simulink model "CF009A_GmOvrlStMgr"  (R2013b)
settings: Solver=FixedStepDiscrete  SolverMode=SingleTasking  StartTime=0.0  StopTime=1  FixedStep=0.002  RelTol=1e-3
values from neighbouring files (symbols this model uses):
  APASTACTV_CNT_U08 = DataDict.Constant    [CF009A_GmOvrlStMgr_DataDict.m]
  APASTCTRLAVL_CNT_U08 = DataDict.Constant    [CF009A_GmOvrlStMgr_DataDict.m]
  ARCHGLBPRM_2MILLISEC_SEC_F32 = DataDict.Constant    [CF009A_GmOvrlStMgr_DataDict.m]
  GmOvrlStMgrApaHwTqThd = DataDict.Calibration    [CF009A_GmOvrlStMgr_DataDict.m]
  GmOvrlStMgrApaHwTqTiThd = DataDict.Calibration    [CF009A_GmOvrlStMgr_DataDict.m]
  GmOvrlStMgrApaMfgEna = DataDict.Calibration    [CF009A_GmOvrlStMgr_DataDict.m]
  GmOvrlStMgrEscMfgEna = DataDict.Calibration    [CF009A_GmOvrlStMgr_DataDict.m]
  GmOvrlStMgrHaptcAmp = DataDict.Calibration    [CF009A_GmOvrlStMgr_DataDict.m]
  GmOvrlStMgrHaptcDurn = DataDict.Calibration    [CF009A_GmOvrlStMgr_DataDict.m]
  GmOvrlStMgrHaptcFrq = DataDict.Calibration    [CF009A_GmOvrlStMgr_DataDict.m]
  GmOvrlStMgrHaptcReactnTi = DataDict.Calibration    [CF009A_GmOvrlStMgr_DataDict.m]
  GmOvrlStMgrHaptcReqTiThd = DataDict.Calibration    [CF009A_GmOvrlStMgr_DataDict.m]
  GmOvrlStMgrHwAgTarLimr = DataDict.Calibration    [CF009A_GmOvrlStMgr_DataDict.m]
  GmOvrlStMgrLkaHwTqThd1 = DataDict.Calibration    [CF009A_GmOvrlStMgr_DataDict.m]
  GmOvrlStMgrLkaHwTqThd2 = DataDict.Calibration    [CF009A_GmOvrlStMgr_DataDict.m]
  GmOvrlStMgrLkaHwTqTiThd1 = DataDict.Calibration    [CF009A_GmOvrlStMgr_DataDict.m]
  GmOvrlStMgrLkaHwTqTiThd2 = DataDict.Calibration    [CF009A_GmOvrlStMgr_DataDict.m]
  GmOvrlStMgrLkaMfgEna = DataDict.Calibration    [CF009A_GmOvrlStMgr_DataDict.m]
  GmOvrlStMgrLoaMtgtnHaptcFbOffTi = DataDict.Calibration    [CF009A_GmOvrlStMgr_DataDict.m]
  GmOvrlStMgrLoaMtgtnHaptcFbOnTi = DataDict.Calibration    [CF009A_GmOvrlStMgr_DataDict.m]
  GmOvrlStMgrLoaMtgtnHaptcFbStrtOnTi = DataDict.Calibration    [CF009A_GmOvrlStMgr_DataDict.m]
  GmOvrlStMgrLoaMtgtnHaptcFbTqMax = DataDict.Calibration    [CF009A_GmOvrlStMgr_DataDict.m]
  GmOvrlStMgrLoaMtgtnHaptcFbTqMin = DataDict.Calibration    [CF009A_GmOvrlStMgr_DataDict.m]
  GmOvrlStMgrLoaMtgtnHaptcFbVehSpdMax = DataDict.Calibration    [CF009A_GmOvrlStMgr_DataDict.m]
  GmOvrlStMgrLoaMtgtnHaptcFbVehSpdMin = DataDict.Calibration    [CF009A_GmOvrlStMgr_DataDict.m]
  GmOvrlStMgrLoaMtgtnHaptcFrq = DataDict.Calibration    [CF009A_GmOvrlStMgr_DataDict.m]
  GmOvrlStMgrLoaMtgtnStrtHaptcAmp = DataDict.Calibration    [CF009A_GmOvrlStMgr_DataDict.m]
  GmOvrlStMgrLoaStIgnCntrThd = DataDict.Calibration    [CF009A_GmOvrlStMgr_DataDict.m]
  GmOvrlStMgrShiftLvrTiThd = DataDict.Calibration    [CF009A_GmOvrlStMgr_DataDict.m]
  GmOvrlStMgrStandStillThd = DataDict.Calibration    [CF009A_GmOvrlStMgr_DataDict.m]
  GmOvrlStMgrStandStillTiThd = DataDict.Calibration    [CF009A_GmOvrlStMgr_DataDict.m]
  HAPTCSTACTV_CNT_U08 = DataDict.Constant    [CF009A_GmOvrlStMgr_DataDict.m]
  HAPTCSTWAIT_CNT_U08 = DataDict.Constant    [CF009A_GmOvrlStMgr_DataDict.m]
  HWOSCNFRQMIN_HZ_F32 = DataDict.Constant    [CF009A_GmOvrlStMgr_DataDict.m]
  LKAFLTCNTRTHD_CNT_U08 = DataDict.Constant    [CF009A_GmOvrlStMgr_DataDict.m]
  LKAFLTTMRTHD_MILLISEC_U32 = DataDict.Constant    [CF009A_GmOvrlStMgr_DataDict.m]
  LKASTPRMNTFAILD_CNT_U08 = DataDict.Constant    [CF009A_GmOvrlStMgr_DataDict.m]
  LoaMtgtnThdExcdd = DataDict.NTC    [CF009A_GmOvrlStMgr_DataDict.m]
  MILLISECTO100MICROSECCNVN_CNT_U32 = DataDict.Constant    [CF009A_GmOvrlStMgr_DataDict.m]
  NODEBSTEP_CNT_U16 = DataDict.Constant    [CF009A_GmOvrlStMgr_DataDict.m]
undefined symbols (not defined in the file or in its folder): LoaSt1, NtcSts1, NVM_RequestResultType, SysSt1
libraries: simulink x13, Fil x6, NxtrNvM x4, NxtrLim x4, NxtrAbslt x3, NxtrSign x2, FixdToFloat x1, FloatToFixd x1, LnrIntrpn x1
(part 4 of 8)

== system CF009A_GmOvrlStMgr/GmOvrlStMgr/GmOvrlStMgrPer1/Inct_IgnCntr_Once/IgnCntr ==
  IgnCntrLcl : Inport  RequirementInfo={} %GIDa_40254b48_8d20_47a3_99f1_0af0fba286b0
  Action Port : ActionPort  InitializeStates=reset  ActionType=then
  Add : Sum
  Constant1 : Constant  Value=true  OutDataTypeStr=boolean
      settings: AttributesFormatString=%<OutDataTypeStr>
  Constant7 : Constant  Value=true  OutDataTypeStr=boolean
      settings: AttributesFormatString=%<OutDataTypeStr>
  Constant8 : Constant  OutDataTypeStr=Inherit: Inherit via back propagation
  CopyRight2 : Subsystem  Description=|  mask(Copyright Information){none=on}
      | Copyright info block.                                               
      |                                                                     
      | Place copyright information at the top of every subsystem in design.
      mask prompts: none "No parameters"
      mask help: Place copyright information at the top of every subsystem in design.
      mask Display:
      | NxtrConf = 'Nexteer Confidential';
      | 
      | sys = bdroot; %handle for the current model ("system")
      | first = get_param(sys,'Created');
      | if(isempty(first))
      |     first = datestr(now,'yyyy');
      | else
      |     first = first(end-3:end);  %year is last four digits
      | end
      | 
      | last = get_param(sys,'LastModifiedDate');
      | if isempty(last)
      |     last = datestr(now,'yyyy');
      | else
      |     last = last(end-3:end);
      | end
      | 
      | if strcmp(first,last)
      |     fprintf('%s -- Copyright %s Nexteer',NxtrConf,first)
      | else
      |     fprintf('%s -- %s%s- %s Nexteer',NxtrConf,char(169),first,last)
      | end
  Data Store Write7 : DataStoreWrite  DataStoreName=IgnCntrUpd
  Data Store Write9 : DataStoreWrite  DataStoreName=GmLoaIgnCntr
  GmLoaIgnCntr_Set Ram Block Status : NxtrNvM/Set Ram Block Status  FuncName=Set Ram Block Status  NvMBlockName=GmLoaIgnCntr  VoidFuncRtn=on  BlockChanged_DSN=NvMSRBS_BlockChanged  Return_DSN=NvMSRBS_Return
      settings: AttributesFormatString=%<FuncName>
  wires:
  Constant8/1 -> Add/2
  IgnCntrLcl/1 -> Add/1
  Add/1 -> Data Store Write9/1
  Constant7/1 -> Data Store Write7/1
  Constant1/1 -> GmLoaIgnCntr_Set Ram Block Status/1

== system CF009A_GmOvrlStMgr/GmOvrlStMgr/GmOvrlStMgrPer1/LKAIntv/CopyRight2 ==

== system CF009A_GmOvrlStMgr/GmOvrlStMgr/GmOvrlStMgrPer1/LKAIntv/HwTqLkaTqSignEqu ==
  Action Port : ActionPort  ActionType=then
  Constant13 : Constant  RequirementInfo={} %GIDa_343d1ac2_1708_4e02_a600_9208d3bcc3bc  Value=false  OutDataTypeStr=boolean
      settings: AttributesFormatString=%<OutDataTypeStr>
  CopyRight2 : Subsystem  Description=|  mask(Copyright Information){none=on}
      | Copyright info block.                                               
      |                                                                     
      | Place copyright information at the top of every subsystem in design.
      mask prompts: none "No parameters"
      mask help: Place copyright information at the top of every subsystem in design.
      mask Display:
      | NxtrConf = 'Nexteer Confidential';
      | 
      | sys = bdroot; %handle for the current model ("system")
      | first = get_param(sys,'Created');
      | first = first(end-3:end);  %year is last four digits
      | 
      | last = get_param(sys,'LastModifiedDate');
      | if isempty(last)
      |     last = datestr(now,'yyyy');
      | else
      |     last = last(end-3:end);
      | end
      | 
      | if strcmp(first,last)
      |     fprintf('%s -- Copyright %s Nexteer',NxtrConf,first)
      | else
      |     fprintf('%s -- %s%s- %s Nexteer',NxtrConf,char(169),first,last)
      | end
  Data Store Write1 : DataStoreWrite  DataStoreName=LkaIntvRefTi2
  Data Store Write9 : DataStoreWrite  DataStoreName=LkaIntvRefTi1
  GetRefTmr100MicroSec32bit : Subsystem
  GetRefTmr100MicroSec32bit_1 : Subsystem
  LKAIntv : Outport
  wires:
  Constant13/1 -> LKAIntv/1
  GetRefTmr100MicroSec32bit/1(RefTmr) -> Data Store Write9/1
  GetRefTmr100MicroSec32bit_1/1(RefTmr) -> Data Store Write1/1

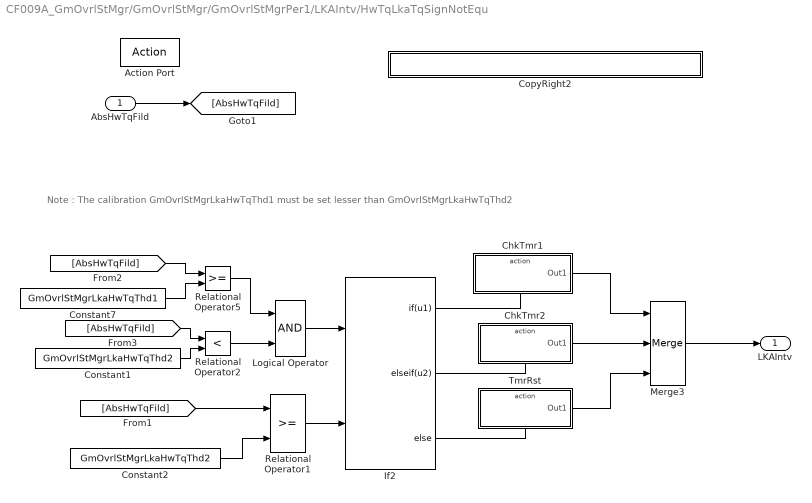
== system CF009A_GmOvrlStMgr/GmOvrlStMgr/GmOvrlStMgrPer1/LKAIntv/HwTqLkaTqSignNotEqu ==
  note: Note : The calibration GmOvrlStMgrLkaHwTqThd1 must be set lesser than GmOvrlStMgrLkaHwTqThd2
  AbsHwTqFild : Inport
  Action Port : ActionPort  ActionType=else
  ChkTmr1 : Subsystem  TreatAsAtomicUnit=on
  ChkTmr2 : Subsystem  TreatAsAtomicUnit=on
  Constant1 : Constant  Value=GmOvrlStMgrLkaHwTqThd2
  Constant2 : Constant  Value=GmOvrlStMgrLkaHwTqThd2
  Constant7 : Constant  Value=GmOvrlStMgrLkaHwTqThd1
  CopyRight2 : Subsystem  Description=|  mask(Copyright Information){none=on}
      | Copyright info block.                                               
      |                                                                     
      | Place copyright information at the top of every subsystem in design.
      mask prompts: none "No parameters"
      mask help: Place copyright information at the top of every subsystem in design.
      mask Display:
      | NxtrConf = 'Nexteer Confidential';
      | 
      | sys = bdroot; %handle for the current model ("system")
      | first = get_param(sys,'Created');
      | first = first(end-3:end);  %year is last four digits
      | 
      | last = get_param(sys,'LastModifiedDate');
      | if isempty(last)
      |     last = datestr(now,'yyyy');
      | else
      |     last = last(end-3:end);
      | end
      | 
      | if strcmp(first,last)
      |     fprintf('%s -- Copyright %s Nexteer',NxtrConf,first)
      | else
      |     fprintf('%s -- %s%s- %s Nexteer',NxtrConf,char(169),first,last)
      | end
  If2 : If  NumInputs=2  IfExpression=u1  ElseIfExpressions=u2
  Logical Operator : Logic  AllPortsSameDT=off  OutDataTypeStr=boolean
  Merge3 : Merge  Inputs=3
  Relational Operator1 : RelationalOperator  OutDataTypeStr=boolean
  Relational Operator2 : RelationalOperator  Operator=<  OutDataTypeStr=boolean
  Relational Operator5 : RelationalOperator  OutDataTypeStr=boolean
  TmrRst : Subsystem  TreatAsAtomicUnit=on
  LKAIntv : Outport
  wires:
  Logical Operator/1 -> If2/1
  Constant7/1 -> Relational Operator5/2
  [AbsHwTqFild] -> Relational Operator1/1
  Relational Operator1/1 -> If2/2
  Constant2/1 -> Relational Operator1/2
  If2/1 -> ChkTmr1/Action
  If2/2 -> ChkTmr2/Action
  If2/3 -> TmrRst/Action
  AbsHwTqFild/1 -> [AbsHwTqFild]
  [AbsHwTqFild] -> Relational Operator5/1
  ChkTmr2/1(Out1) -> Merge3/2
  ChkTmr1/1(Out1) -> Merge3/1
  TmrRst/1(Out1) -> Merge3/3
  Constant1/1 -> Relational Operator2/2
  [AbsHwTqFild] -> Relational Operator2/1
  Relational Operator5/1 -> Logical Operator/1
  Relational Operator2/1 -> Logical Operator/2
  Merge3/1 -> LKAIntv/1

== system CF009A_GmOvrlStMgr/GmOvrlStMgr/GmOvrlStMgrPer1/LkaCheck/CopyRight1 ==

== system CF009A_GmOvrlStMgr/GmOvrlStMgr/GmOvrlStMgrPer1/LkaCheck/CopyRight2 ==

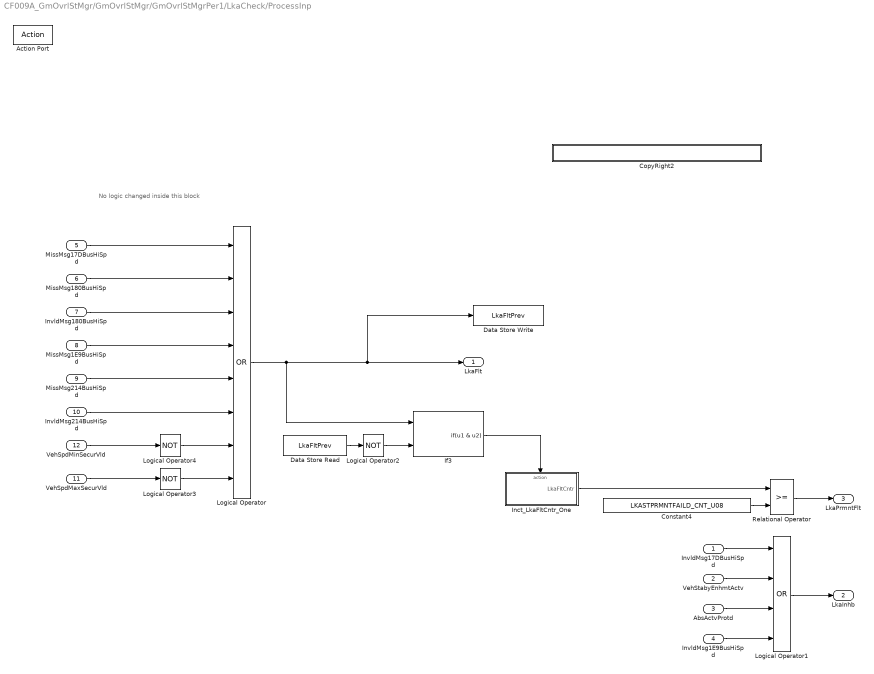
== system CF009A_GmOvrlStMgr/GmOvrlStMgr/GmOvrlStMgrPer1/LkaCheck/ProcessInp ==
  note: No logic changed inside this block
  InvldMsg17DBusHiSpd : Inport  RequirementInfo={} %GIDa_ab38f364_fb54_43ac_97fb_df178091b6c1
  VehStabyEnhmtActv : Inport  RequirementInfo={} %GIDa_14faf567_e873_4922_a66e_aab04f66d7c3  Port=2
  AbsActvProtd : Inport  RequirementInfo={} %GIDa_a55d01c1_013b_4525_9432_b498c288d3b3  Port=3
  InvldMsg1E9BusHiSpd : Inport  RequirementInfo={} %GIDa_3ed3612c_6ee8_4a1a_b952_8a9e955ddcf1  Port=4
  MissMsg17DBusHiSpd : Inport  RequirementInfo={} %GIDa_e64a72e9_2517_49f8_a6e5_489273597452  Port=5
  MissMsg180BusHiSpd : Inport  RequirementInfo={} %GIDa_2fabbd9a_4f5e_4808_82cc_2e9f3cd02a49  Port=6
  InvldMsg180BusHiSpd : Inport  RequirementInfo={} %GIDa_322da83d_5a43_4b7c_bcd7_98015d045729  Port=7
  MissMsg1E9BusHiSpd : Inport  RequirementInfo={} %GIDa_13222ae9_8796_4dca_b882_a83b9d93d3cb  Port=8
  MissMsg214BusHiSpd : Inport  RequirementInfo={} %GIDa_1bf44673_30db_49ae_bdac_03d5de220bff  Port=9
  InvldMsg214BusHiSpd : Inport  RequirementInfo={} %GIDa_9d83abc3_8b94_4471_9b6e_3a35c366fb39  Port=10
  VehSpdMaxSecurVld : Inport  Port=11
  VehSpdMinSecurVld : Inport  Port=12
  Action Port : ActionPort  ActionType=then
  Constant4 : Constant  RequirementInfo={} %GIDa_94974dc5_adaa_4b71_913a_ea3d1a9969a7  Value=LKASTPRMNTFAILD_CNT_U08
  CopyRight2 : Subsystem  Description=|  mask(Copyright Information){none=on}
      | Copyright info block.                                               
      |                                                                     
      | Place copyright information at the top of every subsystem in design.
      mask prompts: none "No parameters"
      mask help: Place copyright information at the top of every subsystem in design.
      mask Display:
      | NxtrConf = 'Nexteer Confidential';
      | 
      | sys = bdroot; %handle for the current model ("system")
      | first = get_param(sys,'Created');
      | if(isempty(first))
      |     first = datestr(now,'yyyy');
      | else
      |     first = first(end-3:end);  %year is last four digits
      | end
      | 
      | last = get_param(sys,'LastModifiedDate');
      | if isempty(last)
      |     last = datestr(now,'yyyy');
      | else
      |     last = last(end-3:end);
      | end
      | 
      | if strcmp(first,last)
      |     fprintf('%s -- Copyright %s Nexteer',NxtrConf,first)
      | else
      |     fprintf('%s -- %s%s- %s Nexteer',NxtrConf,char(169),first,last)
      | end
  Data Store Read : DataStoreRead  Priority=1  DataStoreName=LkaFltPrev
      settings: AttributesFormatString=Priority: %<Priority>
  Data Store Write : DataStoreWrite  Priority=2  DataStoreName=LkaFltPrev
      settings: AttributesFormatString=Priority: %<Priority>
  If3 : If  NumInputs=2  IfExpression=u1 & u2  ShowElse=off
  Inct_LkaFltCntr_One : Subsystem
  Logical Operator : Logic  Operator=OR  Inputs=8  AllPortsSameDT=off  OutDataTypeStr=boolean
  Logical Operator1 : Logic  Operator=OR  Inputs=4  AllPortsSameDT=off  OutDataTypeStr=boolean
  Logical Operator2 : Logic  Operator=NOT  AllPortsSameDT=off  OutDataTypeStr=boolean
  Logical Operator3 : Logic  Operator=NOT  AllPortsSameDT=off  OutDataTypeStr=boolean
  Logical Operator4 : Logic  Operator=NOT  AllPortsSameDT=off  OutDataTypeStr=boolean
  Relational Operator : RelationalOperator  OutDataTypeStr=boolean
  LkaFlt : Outport
  LkaInhb : Outport  Port=2
  LkaPrmntFlt : Outport  Port=3
  wires:
  Relational Operator/1 -> LkaPrmntFlt/1
  Logical Operator1/1 -> LkaInhb/1
  Constant4/1 -> Relational Operator/2
  MissMsg17DBusHiSpd/1 -> Logical Operator/1
  MissMsg180BusHiSpd/1 -> Logical Operator/2
  InvldMsg180BusHiSpd/1 -> Logical Operator/3
  MissMsg1E9BusHiSpd/1 -> Logical Operator/4
  MissMsg214BusHiSpd/1 -> Logical Operator/5
  InvldMsg214BusHiSpd/1 -> Logical Operator/6
  InvldMsg17DBusHiSpd/1 -> Logical Operator1/1
  VehStabyEnhmtActv/1 -> Logical Operator1/2
  AbsActvProtd/1 -> Logical Operator1/3
  InvldMsg1E9BusHiSpd/1 -> Logical Operator1/4
  Logical Operator/1 -> If3/1, Data Store Write/1, LkaFlt/1
  If3/1 -> Inct_LkaFltCntr_One/Action
  Inct_LkaFltCntr_One/1(LkaFltCntr) -> Relational Operator/1
  VehSpdMinSecurVld/1 -> Logical Operator4/1
  VehSpdMaxSecurVld/1 -> Logical Operator3/1
  Data Store Read/1 -> Logical Operator2/1
  Logical Operator2/1 -> If3/2
  Logical Operator3/1 -> Logical Operator/8
  Logical Operator4/1 -> Logical Operator/7

== system CF009A_GmOvrlStMgr/GmOvrlStMgr/GmOvrlStMgrPer1/LkaCheck/SetDefVal ==
  Action Port : ActionPort  ActionType=else
  Constant1 : Constant  Value=0  OutDataTypeStr=boolean
      settings: AttributesFormatString=%<OutDataTypeStr>
  Constant2 : Constant  Value=0  OutDataTypeStr=boolean
      settings: AttributesFormatString=%<OutDataTypeStr>
  Constant6 : Constant  Value=0  OutDataTypeStr=boolean
      settings: AttributesFormatString=%<OutDataTypeStr>
  CopyRight2 : Subsystem  Description=|  mask(Copyright Information){none=on}
      | Copyright info block.                                               
      |                                                                     
      | Place copyright information at the top of every subsystem in design.
      mask prompts: none "No parameters"
      mask help: Place copyright information at the top of every subsystem in design.
      mask Display:
      | NxtrConf = 'Nexteer Confidential';
      | 
      | sys = bdroot; %handle for the current model ("system")
      | first = get_param(sys,'Created');
      | if(isempty(first))
      |     first = datestr(now,'yyyy');
      | else
      |     first = first(end-3:end);  %year is last four digits
      | end
      | 
      | last = get_param(sys,'LastModifiedDate');
      | if isempty(last)
      |     last = datestr(now,'yyyy');
      | else
      |     last = last(end-3:end);
      | end
      | 
      | if strcmp(first,last)
      |     fprintf('%s -- Copyright %s Nexteer',NxtrConf,first)
      | else
      |     fprintf('%s -- %s%s- %s Nexteer',NxtrConf,char(169),first,last)
      | end
  LkaFlt : Outport
  LkaInhb : Outport  Port=2
  LkaPrmntFlt : Outport  Port=3
  wires:
  Constant6/1 -> LkaFlt/1
  Constant1/1 -> LkaInhb/1
  Constant2/1 -> LkaPrmntFlt/1

== system CF009A_GmOvrlStMgr/GmOvrlStMgr/GmOvrlStMgrPer1/LkaCheck/TmrElpdDetn ==
  LkaFltRefTmr : Inport
  Constant : Constant  Value=LKAFLTTMRTHD_MILLISEC_U32
  Constant1 : Constant  Value=MILLISECTO100MICROSECCNVN_CNT_U32
  CopyRight2 : Subsystem  Description=|  mask(Copyright Information){none=on}
      | Copyright info block.                                               
      |                                                                     
      | Place copyright information at the top of every subsystem in design.
      mask prompts: none "No parameters"
      mask help: Place copyright information at the top of every subsystem in design.
      mask Display:
      | NxtrConf = 'Nexteer Confidential';
      | 
      | sys = bdroot; %handle for the current model ("system")
      | first = get_param(sys,'Created');
      | if(isempty(first))
      |     first = datestr(now,'yyyy');
      | else
      |     first = first(end-3:end);  %year is last four digits
      | end
      | 
      | last = get_param(sys,'LastModifiedDate');
      | if isempty(last)
      |     last = datestr(now,'yyyy');
      | else
      |     last = last(end-3:end);
      | end
      | 
      | if strcmp(first,last)
      |     fprintf('%s -- Copyright %s Nexteer',NxtrConf,first)
      | else
      |     fprintf('%s -- %s%s- %s Nexteer',NxtrConf,char(169),first,last)
      | end
  GetTiSpan100MicroSec32bit : Subsystem
  Product : Product
  Relational Operator : RelationalOperator  OutDataTypeStr=boolean
  TiElpd : Outport
  wires:
  LkaFltRefTmr/1 -> GetTiSpan100MicroSec32bit/1(RefTmr)
  GetTiSpan100MicroSec32bit/1(TiSpan) -> Relational Operator/1
  Product/1 -> Relational Operator/2
  Constant/1 -> Product/1
  Constant1/1 -> Product/2
  Relational Operator/1 -> TiElpd/1

== system CF009A_GmOvrlStMgr/GmOvrlStMgr/GmOvrlStMgrPer1/LoaStLimdOrSwBasdMtgtn/CopyRight2 ==

== system CF009A_GmOvrlStMgr/GmOvrlStMgr/GmOvrlStMgrPer1/LoaStLimdOrSwBasdMtgtn/Set_false_LoaStLimdOrSwBasdMtgtn ==
  Action Port : ActionPort  ActionType=else
  Constant2 : Constant  Value=false  OutDataTypeStr=boolean
      settings: AttributesFormatString=%<OutDataTypeStr>
  CopyRight2 : Subsystem  Description=|  mask(Copyright Information){none=on}
      | Copyright info block.                                               
      |                                                                     
      | Place copyright information at the top of every subsystem in design.
      mask prompts: none "No parameters"
      mask help: Place copyright information at the top of every subsystem in design.
      mask Display:
      | NxtrConf = 'Nexteer Confidential';
      | 
      | sys = bdroot; %handle for the current model ("system")
      | first = get_param(sys,'Created');
      | if(isempty(first))
      |     first = datestr(now,'yyyy');
      | else
      |     first = first(end-3:end);  %year is last four digits
      | end
      | 
      | last = get_param(sys,'LastModifiedDate');
      | if isempty(last)
      |     last = datestr(now,'yyyy');
      | else
      |     last = last(end-3:end);
      | end
      | 
      | if strcmp(first,last)
      |     fprintf('%s -- Copyright %s Nexteer',NxtrConf,first)
      | else
      |     fprintf('%s -- %s%s- %s Nexteer',NxtrConf,char(169),first,last)
      | end
  LoaStLimdOrSwBasdMtgtn : Outport
  wires:
  Constant2/1 -> LoaStLimdOrSwBasdMtgtn/1

== system CF009A_GmOvrlStMgr/GmOvrlStMgr/GmOvrlStMgrPer1/LoaStLimdOrSwBasdMtgtn/Set_true_LoaStLimdOrSwBasdMtgtn ==
  Action Port : ActionPort  ActionType=then
  Constant2 : Constant  Value=true  OutDataTypeStr=boolean
      settings: AttributesFormatString=%<OutDataTypeStr>
  CopyRight2 : Subsystem  Description=|  mask(Copyright Information){none=on}
      | Copyright info block.                                               
      |                                                                     
      | Place copyright information at the top of every subsystem in design.
      mask prompts: none "No parameters"
      mask help: Place copyright information at the top of every subsystem in design.
      mask Display:
      | NxtrConf = 'Nexteer Confidential';
      | 
      | sys = bdroot; %handle for the current model ("system")
      | first = get_param(sys,'Created');
      | if(isempty(first))
      |     first = datestr(now,'yyyy');
      | else
      |     first = first(end-3:end);  %year is last four digits
      | end
      | 
      | last = get_param(sys,'LastModifiedDate');
      | if isempty(last)
      |     last = datestr(now,'yyyy');
      | else
      |     last = last(end-3:end);
      | end
      | 
      | if strcmp(first,last)
      |     fprintf('%s -- Copyright %s Nexteer',NxtrConf,first)
      | else
      |     fprintf('%s -- %s%s- %s Nexteer',NxtrConf,char(169),first,last)
      | end
  LoaStLimdOrSwBasdMtgtn : Outport
  wires:
  Constant2/1 -> LoaStLimdOrSwBasdMtgtn/1

== system CF009A_GmOvrlStMgr/GmOvrlStMgr/GmOvrlStMgrPer1/SysStNotOperate_TqOscnDi_AmpZero_FrqMin/CopyRight2 ==

== system CF009A_GmOvrlStMgr/GmOvrlStMgr/GmOvrlStMgrPer1/SysStOperate/Chk_LoaSt_IgnCntr_ AtStartUp ==
  IgnCntrLcl : Inport  RequirementInfo={} %GIDa_e8697a3d_ab56_4bb3_bef2_1b8a01945d63
  LoaStLimdOrSwBasdMtgtn : Inport  RequirementInfo={} %GIDa_6f19b0cf_19ed_4211_a8d1_72361d5bd862  Port=2
  Action Port : ActionPort  ActionType=then
  Constant5 : Constant  Value=GmOvrlStMgrLoaStIgnCntrThd
  CopyRight2 : Subsystem  Description=|  mask(Copyright Information){none=on}
      | Copyright info block.                                               
      |                                                                     
      | Place copyright information at the top of every subsystem in design.
      mask prompts: none "No parameters"
      mask help: Place copyright information at the top of every subsystem in design.
      mask Display:
      | NxtrConf = 'Nexteer Confidential';
      | 
      | sys = bdroot; %handle for the current model ("system")
      | first = get_param(sys,'Created');
      | if(isempty(first))
      |     first = datestr(now,'yyyy');
      | else
      |     first = first(end-3:end);  %year is last four digits
      | end
      | 
      | last = get_param(sys,'LastModifiedDate');
      | if isempty(last)
      |     last = datestr(now,'yyyy');
      | else
      |     last = last(end-3:end);
      | end
      | 
      | if strcmp(first,last)
      |     fprintf('%s -- Copyright %s Nexteer',NxtrConf,first)
      | else
      |     fprintf('%s -- %s%s- %s Nexteer',NxtrConf,char(169),first,last)
      | end
  HaptcFbOn : Subsystem  TreatAsAtomicUnit=on
  If4 : If  NumInputs=2  IfExpression=u1&u2
  Merge1 : Merge
  Merge2 : Merge
  Merge3 : Merge
  Relational Operator5 : RelationalOperator  Operator=<  OutDataTypeStr=boolean
  Set_True_LoaStAlreadyChk_HaptcFbOff : Subsystem  TreatAsAtomicUnit=on
  HaptcFbEn : Outport
  HwOscnMotAmp : Outport  RequirementInfo={} %GIDa_94979410_e9f4_4c1d_b419_ebbe160cd395  Port=2
  HwOscnFrq : Outport  RequirementInfo={} %GIDa_7e58c67f_3cab_4a1d_80f1_5b93bb1627c0  Port=3
  wires:
  If4/1 -> HaptcFbOn/Action
  If4/2 -> Set_True_LoaStAlreadyChk_HaptcFbOff/Action
  HaptcFbOn/2(HwOscnMotAmp) -> Merge1/1
  HaptcFbOn/1(HaptcFbEn) -> Merge2/1
  HaptcFbOn/3(HwOscnFrq) -> Merge3/1
  Set_True_LoaStAlreadyChk_HaptcFbOff/1(HwOscnEna) -> Merge2/2
  Set_True_LoaStAlreadyChk_HaptcFbOff/3(HwOscnFrq) -> Merge3/2
  Set_True_LoaStAlreadyChk_HaptcFbOff/2(HwOscnMotAmp) -> Merge1/2
  Merge2/1 -> HaptcFbEn/1
  Merge3/1 -> HwOscnFrq/1
  Merge1/1 -> HwOscnMotAmp/1
  Constant5/1 -> Relational Operator5/2
  IgnCntrLcl/1 -> Relational Operator5/1
  Relational Operator5/1 -> If4/1
  LoaStLimdOrSwBasdMtgtn/1 -> If4/2

== system CF009A_GmOvrlStMgr/GmOvrlStMgr/GmOvrlStMgrPer1/SysStOperate/CopyRight2 ==

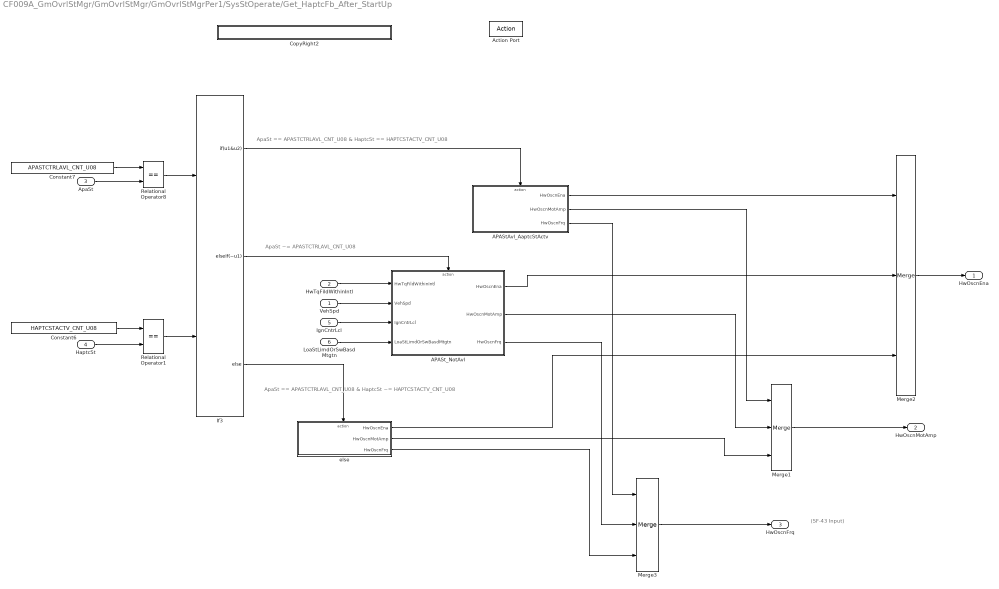
== system CF009A_GmOvrlStMgr/GmOvrlStMgr/GmOvrlStMgrPer1/SysStOperate/Get_HaptcFb_After_StartUp ==
  note: ApaSt == APASTCTRLAVL_CNT_U08 & HaptcSt ~= HAPTCSTACTV_CNT_U08
  note: ApaSt ~= APASTCTRLAVL_CNT_U08
  note: ApaSt == APASTCTRLAVL_CNT_U08 & HaptcSt == HAPTCSTACTV_CNT_U08
  note: (SF-43 Input)
  VehSpd : Inport  RequirementInfo={} %GIDa_a5829b81_07ba_4c64_8787_8fc04ee14cfd
  HwTqFildWithinIntl : Inport  RequirementInfo={} %GIDa_e61ff016_f3ba_4ff0_a83d_54857dcede2c  Port=2
  ApaSt : Inport  RequirementInfo={} %GIDa_e54ff0fb_14e3_45e1_9566_d1512fd62416  Port=3
  HaptcSt : Inport  RequirementInfo={} %GIDa_ab8a4f54_44b6_4424_b05e_8238140c4b6c  Port=4
  IgnCntrLcl : Inport  RequirementInfo={} %GIDa_b0910f28_8214_48fc_9951_e54f19ad46d2  Port=5
  LoaStLimdOrSwBasdMtgtn : Inport  RequirementInfo={} %GIDa_58f7fd75_e089_4fe4_9a52_37c69388915c  Port=6
  Action Port : ActionPort  ActionType=else
  APAStAvl_AaptcStActv : Subsystem
  APASt_NotAvl : Subsystem
  Constant6 : Constant  RequirementInfo={} %GIDa_58d35ea2_589d_40a1_bd0e_f64c7e93a79e  Value=HAPTCSTACTV_CNT_U08
  Constant7 : Constant  Value=APASTCTRLAVL_CNT_U08
  CopyRight2 : Subsystem  Description=|  mask(Copyright Information){none=on}
      | Copyright info block.                                               
      |                                                                     
      | Place copyright information at the top of every subsystem in design.
      mask prompts: none "No parameters"
      mask help: Place copyright information at the top of every subsystem in design.
      mask Display:
      | NxtrConf = 'Nexteer Confidential';
      | 
      | sys = bdroot; %handle for the current model ("system")
      | first = get_param(sys,'Created');
      | if(isempty(first))
      |     first = datestr(now,'yyyy');
      | else
      |     first = first(end-3:end);  %year is last four digits
      | end
      | 
      | last = get_param(sys,'LastModifiedDate');
      | if isempty(last)
      |     last = datestr(now,'yyyy');
      | else
      |     last = last(end-3:end);
      | end
      | 
      | if strcmp(first,last)
      |     fprintf('%s -- Copyright %s Nexteer',NxtrConf,first)
      | else
      |     fprintf('%s -- %s%s- %s Nexteer',NxtrConf,char(169),first,last)
      | end
  If3 : If  NumInputs=2  IfExpression=u1&u2  ElseIfExpressions=~u1
  Merge1 : Merge  Inputs=3
  Merge2 : Merge  Inputs=3
  Merge3 : Merge  Inputs=3
  Relational Operator1 : RelationalOperator  Operator===  OutDataTypeStr=boolean
  Relational Operator8 : RelationalOperator  Operator===  OutDataTypeStr=boolean
  else : Subsystem
  HwOscnEna : Outport  RequirementInfo={} %GIDa_60abaf6a_645d_41f4_bc17_5a7267f09745
  HwOscnMotAmp : Outport  RequirementInfo={} %GIDa_33c54218_d95c_4bd4_ac09_6c51a9d1e98a  Port=2
  HwOscnFrq : Outport  RequirementInfo={} %GIDa_08ffb019_6499_48c1_85d5_d35ae98c4cad  Port=3
  wires:
  VehSpd/1 -> APASt_NotAvl/2(VehSpd)
  Relational Operator1/1 -> If3/2
  Constant6/1 -> Relational Operator1/1
  Relational Operator8/1 -> If3/1
  If3/1 -> APAStAvl_AaptcStActv/Action
  If3/3 -> else/Action
  If3/2 -> APASt_NotAvl/Action
  Merge1/1 -> HwOscnMotAmp/1
  Merge3/1 -> HwOscnFrq/1
  APAStAvl_AaptcStActv/1(HwOscnEna) -> Merge2/1
  APASt_NotAvl/1(HwOscnEna) -> Merge2/2
  else/1(HwOscnEna) -> Merge2/3
  APAStAvl_AaptcStActv/2(HwOscnMotAmp) -> Merge1/1
  APASt_NotAvl/2(HwOscnMotAmp) -> Merge1/2
  else/2(HwOscnMotAmp) -> Merge1/3
  APAStAvl_AaptcStActv/3(HwOscnFrq) -> Merge3/1
  APASt_NotAvl/3(HwOscnFrq) -> Merge3/2
  else/3(HwOscnFrq) -> Merge3/3
  Merge2/1 -> HwOscnEna/1
  HwTqFildWithinIntl/1 -> APASt_NotAvl/1(HwTqFildWithinIntl)
  HaptcSt/1 -> Relational Operator1/2
  Constant7/1 -> Relational Operator8/1
  ApaSt/1 -> Relational Operator8/2
  IgnCntrLcl/1 -> APASt_NotAvl/3(IgnCntrLcl)
  LoaStLimdOrSwBasdMtgtn/1 -> APASt_NotAvl/4(LoaStLimdOrSwBasdMtgtn)

== system CF009A_GmOvrlStMgr/GmOvrlStMgr/GmOvrlStMgrPer1/Timer for HwHaptcEna/CopyRight2 ==

== system CF009A_GmOvrlStMgr/GmOvrlStMgr/GmOvrlStMgrPer1/Timer for HwHaptcEna/If Action Subsystem ==
  Action Port : ActionPort  ActionType=then
  Constant : Constant  Value=0  OutDataTypeStr=single
  CopyRight2 : Subsystem  Description=|  mask(Copyright Information){none=on}
      | Copyright info block.                                               
      |                                                                     
      | Place copyright information at the top of every subsystem in design.
      mask prompts: none "No parameters"
      mask help: Place copyright information at the top of every subsystem in design.
      mask Display:
      | NxtrConf = 'Nexteer Confidential';
      | 
      | sys = bdroot; %handle for the current model ("system")
      | first = get_param(sys,'Created');
      | if(isempty(first))
      |     first = datestr(now,'yyyy');
      | else
      |     first = first(end-3:end);  %year is last four digits
      | end
      | 
      | last = get_param(sys,'LastModifiedDate');
      | if isempty(last)
      |     last = datestr(now,'yyyy');
      | else
      |     last = last(end-3:end);
      | end
      | 
      | if strcmp(first,last)
      |     fprintf('%s -- Copyright %s Nexteer',NxtrConf,first)
      | else
      |     fprintf('%s -- %s%s- %s Nexteer',NxtrConf,char(169),first,last)
      | end
  Data Store Write : DataStoreWrite  DataStoreName=PrevHaptcReqRefTi
  Data Type Conversion : DataTypeConversion  OutDataTypeStr=uint32
  GetRefTmr100MicroSec32bit : Subsystem
  Out : Outport
  wires:
  Constant/1 -> Data Type Conversion/1
  GetRefTmr100MicroSec32bit/1(RefTmr) -> Data Store Write/1
  Data Type Conversion/1 -> Out/1

== system CF009A_GmOvrlStMgr/GmOvrlStMgr/GmOvrlStMgrPer1/Timer for HwHaptcEna/If Action Subsystem1 ==
  In1 : Inport
  Action Port : ActionPort  ActionType=else
  CopyRight2 : Subsystem  Description=|  mask(Copyright Information){none=on}
      | Copyright info block.                                               
      |                                                                     
      | Place copyright information at the top of every subsystem in design.
      mask prompts: none "No parameters"
      mask help: Place copyright information at the top of every subsystem in design.
      mask Display:
      | NxtrConf = 'Nexteer Confidential';
      | 
      | sys = bdroot; %handle for the current model ("system")
      | first = get_param(sys,'Created');
      | if(isempty(first))
      |     first = datestr(now,'yyyy');
      | else
      |     first = first(end-3:end);  %year is last four digits
      | end
      | 
      | last = get_param(sys,'LastModifiedDate');
      | if isempty(last)
      |     last = datestr(now,'yyyy');
      | else
      |     last = last(end-3:end);
      | end
      | 
      | if strcmp(first,last)
      |     fprintf('%s -- Copyright %s Nexteer',NxtrConf,first)
      | else
      |     fprintf('%s -- %s%s- %s Nexteer',NxtrConf,char(169),first,last)
      | end
  Out1 : Outport
  wires:
  In1/1 -> Out1/1

== system CF009A_GmOvrlStMgr/GmOvrlStMgr/GmOvrlStMgrPer1/Timer for HwHaptcEna/If Action Subsystem2 ==
  Action Port : ActionPort  ActionType=elseif
  CopyRight2 : Subsystem  Description=|  mask(Copyright Information){none=on}
      | Copyright info block.                                               
      |                                                                     
      | Place copyright information at the top of every subsystem in design.
      mask prompts: none "No parameters"
      mask help: Place copyright information at the top of every subsystem in design.
      mask Display:
      | NxtrConf = 'Nexteer Confidential';
      | 
      | sys = bdroot; %handle for the current model ("system")
      | first = get_param(sys,'Created');
      | if(isempty(first))
      |     first = datestr(now,'yyyy');
      | else
      |     first = first(end-3:end);  %year is last four digits
      | end
      | 
      | last = get_param(sys,'LastModifiedDate');
      | if isempty(last)
      |     last = datestr(now,'yyyy');
      | else
      |     last = last(end-3:end);
      | end
      | 
      | if strcmp(first,last)
      |     fprintf('%s -- Copyright %s Nexteer',NxtrConf,first)
      | else
      |     fprintf('%s -- %s%s- %s Nexteer',NxtrConf,char(169),first,last)
      | end
  Data Store Read : DataStoreRead  DataStoreName=PrevHaptcReqRefTi
  GetTiSpan100MicroSec32bit1 : Subsystem
  Out1 : Outport
  wires:
  GetTiSpan100MicroSec32bit1/1(TiSpan) -> Out1/1
  Data Store Read/1 -> GetTiSpan100MicroSec32bit1/1(RefTmr)

== system CF009A_GmOvrlStMgr/GmOvrlStMgr/GmOvrlStMgrPer1/Timer for ShiftLvrRvs/CopyRight2 ==

== system CF009A_GmOvrlStMgr/GmOvrlStMgr/GmOvrlStMgrPer1/Timer for ShiftLvrRvs/If Action Subsystem ==
  Action Port : ActionPort  ActionType=then
  Constant : Constant  Value=0  OutDataTypeStr=single
  CopyRight2 : Subsystem  Description=|  mask(Copyright Information){none=on}
      | Copyright info block.                                               
      |                                                                     
      | Place copyright information at the top of every subsystem in design.
      mask prompts: none "No parameters"
      mask help: Place copyright information at the top of every subsystem in design.
      mask Display:
      | NxtrConf = 'Nexteer Confidential';
      | 
      | sys = bdroot; %handle for the current model ("system")
      | first = get_param(sys,'Created');
      | first = first(end-3:end);  %year is last four digits
      | 
      | last = get_param(sys,'LastModifiedDate');
      | if isempty(last)
      |     last = datestr(now,'yyyy');
      | else
      |     last = last(end-3:end);
      | end
      | 
      | if strcmp(first,last)
      |     fprintf('%s -- Copyright %s Nexteer',NxtrConf,first)
      | else
      |     fprintf('%s -- %s%s- %s Nexteer',NxtrConf,char(169),first,last)
      | end
  Data Store Write : DataStoreWrite  DataStoreName=PrevShiftLvrRvsRefTi
  Data Type Conversion : DataTypeConversion  OutDataTypeStr=uint32
  GetRefTmr100MicroSec32bit : Subsystem
  Out : Outport
  wires:
  Constant/1 -> Data Type Conversion/1
  GetRefTmr100MicroSec32bit/1(RefTmr) -> Data Store Write/1
  Data Type Conversion/1 -> Out/1

== system CF009A_GmOvrlStMgr/GmOvrlStMgr/GmOvrlStMgrPer1/Timer for ShiftLvrRvs/If Action Subsystem1 ==
  In1 : Inport
  Action Port : ActionPort  ActionType=else
  CopyRight2 : Subsystem  Description=|  mask(Copyright Information){none=on}
      | Copyright info block.                                               
      |                                                                     
      | Place copyright information at the top of every subsystem in design.
      mask prompts: none "No parameters"
      mask help: Place copyright information at the top of every subsystem in design.
      mask Display:
      | NxtrConf = 'Nexteer Confidential';
      | 
      | sys = bdroot; %handle for the current model ("system")
      | first = get_param(sys,'Created');
      | first = first(end-3:end);  %year is last four digits
      | 
      | last = get_param(sys,'LastModifiedDate');
      | if isempty(last)
      |     last = datestr(now,'yyyy');
      | else
      |     last = last(end-3:end);
      | end
      | 
      | if strcmp(first,last)
      |     fprintf('%s -- Copyright %s Nexteer',NxtrConf,first)
      | else
      |     fprintf('%s -- %s%s- %s Nexteer',NxtrConf,char(169),first,last)
      | end
  Out1 : Outport
  wires:
  In1/1 -> Out1/1

== system CF009A_GmOvrlStMgr/GmOvrlStMgr/GmOvrlStMgrPer1/Timer for ShiftLvrRvs/If Action Subsystem2 ==
  Action Port : ActionPort  ActionType=elseif
  CopyRight2 : Subsystem  Description=|  mask(Copyright Information){none=on}
      | Copyright info block.                                               
      |                                                                     
      | Place copyright information at the top of every subsystem in design.
      mask prompts: none "No parameters"
      mask help: Place copyright information at the top of every subsystem in design.
      mask Display:
      | NxtrConf = 'Nexteer Confidential';
      | 
      | sys = bdroot; %handle for the current model ("system")
      | first = get_param(sys,'Created');
      | first = first(end-3:end);  %year is last four digits
      | 
      | last = get_param(sys,'LastModifiedDate');
      | if isempty(last)
      |     last = datestr(now,'yyyy');
      | else
      |     last = last(end-3:end);
      | end
      | 
      | if strcmp(first,last)
      |     fprintf('%s -- Copyright %s Nexteer',NxtrConf,first)
      | else
      |     fprintf('%s -- %s%s- %s Nexteer',NxtrConf,char(169),first,last)
      | end
  Data Store Read : DataStoreRead  DataStoreName=PrevShiftLvrRvsRefTi
  GetTiSpan100MicroSec32bit1 : Subsystem
  Out : Outport
  wires:
  GetTiSpan100MicroSec32bit1/1(TiSpan) -> Out/1
  Data Store Read/1 -> GetTiSpan100MicroSec32bit1/1(RefTmr)

== system CF009A_GmOvrlStMgr/GmOvrlStMgr/GmOvrlStMgrPer1/Timer for VehStandStill/CopyRight2 ==

== system CF009A_GmOvrlStMgr/GmOvrlStMgr/GmOvrlStMgrPer1/Timer for VehStandStill/If Action Subsystem ==
  Action Port : ActionPort  ActionType=then
  Constant : Constant  Value=0  OutDataTypeStr=single
  CopyRight2 : Subsystem  Description=|  mask(Copyright Information){none=on}
      | Copyright info block.                                               
      |                                                                     
      | Place copyright information at the top of every subsystem in design.
      mask prompts: none "No parameters"
      mask help: Place copyright information at the top of every subsystem in design.
      mask Display:
      | NxtrConf = 'Nexteer Confidential';
      | 
      | sys = bdroot; %handle for the current model ("system")
      | first = get_param(sys,'Created');
      | first = first(end-3:end);  %year is last four digits
      | 
      | last = get_param(sys,'LastModifiedDate');
      | if isempty(last)
      |     last = datestr(now,'yyyy');
      | else
      |     last = last(end-3:end);
      | end
      | 
      | if strcmp(first,last)
      |     fprintf('%s -- Copyright %s Nexteer',NxtrConf,first)
      | else
      |     fprintf('%s -- %s%s- %s Nexteer',NxtrConf,char(169),first,last)
      | end
  Data Store Write : DataStoreWrite  DataStoreName=PrevVehStandStillRefTi
  Data Type Conversion : DataTypeConversion  OutDataTypeStr=uint32
  GetRefTmr100MicroSec32bit : Subsystem
  Out : Outport
  wires:
  Constant/1 -> Data Type Conversion/1
  GetRefTmr100MicroSec32bit/1(RefTmr) -> Data Store Write/1
  Data Type Conversion/1 -> Out/1

== system CF009A_GmOvrlStMgr/GmOvrlStMgr/GmOvrlStMgrPer1/Timer for VehStandStill/If Action Subsystem1 ==
  In1 : Inport
  Action Port : ActionPort  ActionType=else
  CopyRight2 : Subsystem  Description=|  mask(Copyright Information){none=on}
      | Copyright info block.                                               
      |                                                                     
      | Place copyright information at the top of every subsystem in design.
      mask prompts: none "No parameters"
      mask help: Place copyright information at the top of every subsystem in design.
      mask Display:
      | NxtrConf = 'Nexteer Confidential';
      | 
      | sys = bdroot; %handle for the current model ("system")
      | first = get_param(sys,'Created');
      | first = first(end-3:end);  %year is last four digits
      | 
      | last = get_param(sys,'LastModifiedDate');
      | if isempty(last)
      |     last = datestr(now,'yyyy');
      | else
      |     last = last(end-3:end);
      | end
      | 
      | if strcmp(first,last)
      |     fprintf('%s -- Copyright %s Nexteer',NxtrConf,first)
      | else
      |     fprintf('%s -- %s%s- %s Nexteer',NxtrConf,char(169),first,last)
      | end
  Out1 : Outport
  wires:
  In1/1 -> Out1/1

== system CF009A_GmOvrlStMgr/GmOvrlStMgr/GmOvrlStMgrPer1/Timer for VehStandStill/If Action Subsystem2 ==
  Action Port : ActionPort  ActionType=elseif
  CopyRight2 : Subsystem  Description=|  mask(Copyright Information){none=on}
      | Copyright info block.                                               
      |                                                                     
      | Place copyright information at the top of every subsystem in design.
      mask prompts: none "No parameters"
      mask help: Place copyright information at the top of every subsystem in design.
      mask Display:
      | NxtrConf = 'Nexteer Confidential';
      | 
      | sys = bdroot; %handle for the current model ("system")
      | first = get_param(sys,'Created');
      | first = first(end-3:end);  %year is last four digits
      | 
      | last = get_param(sys,'LastModifiedDate');
      | if isempty(last)
      |     last = datestr(now,'yyyy');
      | else
      |     last = last(end-3:end);
      | end
      | 
      | if strcmp(first,last)
      |     fprintf('%s -- Copyright %s Nexteer',NxtrConf,first)
      | else
      |     fprintf('%s -- %s%s- %s Nexteer',NxtrConf,char(169),first,last)
      | end
  Data Store Read : DataStoreRead  DataStoreName=PrevVehStandStillRefTi
  GetTiSpan100MicroSec32bit1 : Subsystem
  Out1 : Outport
  wires:
  GetTiSpan100MicroSec32bit1/1(TiSpan) -> Out1/1
  Data Store Read/1 -> GetTiSpan100MicroSec32bit1/1(RefTmr)

== system CF009A_GmOvrlStMgr/GmOvrlStMgr/GmOvrlStMgrPer1/TransHaptcsWaitToAPAStActvFlg/CopyRight2 ==

== system CF009A_GmOvrlStMgr/GmOvrlStMgr/GmOvrlStMgrPer1/TransHaptcsWaitToAPAStActvFlg/ElpseTi ==
  Action Port : ActionPort  ActionType=then
  Constant : Constant  RequirementInfo={} %GIDa_dd7f2756_3d28_475b_ad52_d69d68ef3406  Value=GmOvrlStMgrHaptcReactnTi
  Constant1 : Constant  Value=MILLISECTO100MICROSECCNVN_CNT_U32
  CopyRight2 : Subsystem  Description=|  mask(Copyright Information){none=on}
      | Copyright info block.                                               
      |                                                                     
      | Place copyright information at the top of every subsystem in design.
      mask prompts: none "No parameters"
      mask help: Place copyright information at the top of every subsystem in design.
      mask Display:
      | NxtrConf = 'Nexteer Confidential';
      | 
      | sys = bdroot; %handle for the current model ("system")
      | first = get_param(sys,'Created');
      | if(isempty(first))
      |     first = datestr(now,'yyyy');
      | else
      |     first = first(end-3:end);  %year is last four digits
      | end
      | 
      | last = get_param(sys,'LastModifiedDate');
      | if isempty(last)
      |     last = datestr(now,'yyyy');
      | else
      |     last = last(end-3:end);
      | end
      | 
      | if strcmp(first,last)
      |     fprintf('%s -- Copyright %s Nexteer',NxtrConf,first)
      | else
      |     fprintf('%s -- %s%s- %s Nexteer',NxtrConf,char(169),first,last)
      | end
  Data Store Read : DataStoreRead  DataStoreName=TranHaptcWaitToApaStActvRefTi
  GetTiSpan100MicroSec32bit : Subsystem
  If4 : If  IfExpression=u1
  Merge1 : Merge
  Product1 : Product
  Relational Operator : RelationalOperator  OutDataTypeStr=boolean
  Set False Subsystem : Subsystem  TreatAsAtomicUnit=on
  Set True Subsystem : Subsystem  TreatAsAtomicUnit=on
  Out1 : Outport
  wires:
  Data Store Read/1 -> GetTiSpan100MicroSec32bit/1(RefTmr)
  Merge1/1 -> Out1/1
  GetTiSpan100MicroSec32bit/1(TiSpan) -> Relational Operator/1
  Relational Operator/1 -> If4/1
  If4/1 -> Set True Subsystem/Action
  Set True Subsystem/1(Out1) -> Merge1/1
  Set False Subsystem/1(Out1) -> Merge1/2
  If4/2 -> Set False Subsystem/Action
  Constant1/1 -> Product1/2
  Product1/1 -> Relational Operator/2
  Constant/1 -> Product1/1

== system CF009A_GmOvrlStMgr/GmOvrlStMgr/GmOvrlStMgrPer1/TransHaptcsWaitToAPAStActvFlg/RefTi ==
  Action Port : ActionPort  ActionType=else
  Constant13 : Constant  RequirementInfo={} %GIDa_619d356c_ecb5_4941_96a3_4250e680b170  Value=false  OutDataTypeStr=boolean
      settings: AttributesFormatString=%<OutDataTypeStr>
  CopyRight2 : Subsystem  Description=|  mask(Copyright Information){none=on}
      | Copyright info block.                                               
      |                                                                     
      | Place copyright information at the top of every subsystem in design.
      mask prompts: none "No parameters"
      mask help: Place copyright information at the top of every subsystem in design.
      mask Display:
      | NxtrConf = 'Nexteer Confidential';
      | 
      | sys = bdroot; %handle for the current model ("system")
      | first = get_param(sys,'Created');
      | if(isempty(first))
      |     first = datestr(now,'yyyy');
      | else
      |     first = first(end-3:end);  %year is last four digits
      | end
      | 
      | last = get_param(sys,'LastModifiedDate');
      | if isempty(last)
      |     last = datestr(now,'yyyy');
      | else
      |     last = last(end-3:end);
      | end
      | 
      | if strcmp(first,last)
      |     fprintf('%s -- Copyright %s Nexteer',NxtrConf,first)
      | else
      |     fprintf('%s -- %s%s- %s Nexteer',NxtrConf,char(169),first,last)
      | end
  Data Store Write9 : DataStoreWrite  DataStoreName=TranHaptcWaitToApaStActvRefTi
  GetRefTmr100MicroSec32bit : Subsystem
  Out1 : Outport
  wires:
  GetRefTmr100MicroSec32bit/1(RefTmr) -> Data Store Write9/1
  Constant13/1 -> Out1/1

== system CF009A_GmOvrlStMgr/GmOvrlStMgr/GmOvrlStMgrInit1/NTC_Fault1_Set_Faild/SetNtcSts/CopyRight2 ==

== system CF009A_GmOvrlStMgr/GmOvrlStMgr/GmOvrlStMgrInit1/NTC_Fault1_Set_Passd/SetNtcSts/CopyRight2 ==

== system CF009A_GmOvrlStMgr/GmOvrlStMgr/GmOvrlStMgrPer1/ApaIntv/If Action Subsystem/CopyRight2 ==

== system CF009A_GmOvrlStMgr/GmOvrlStMgr/GmOvrlStMgrPer1/ApaIntv/If Action Subsystem1/CopyRight2 ==

== system CF009A_GmOvrlStMgr/GmOvrlStMgr/GmOvrlStMgrPer1/ApaIntv/Timer for ApaIntv/CopyRight2 ==

== system CF009A_GmOvrlStMgr/GmOvrlStMgr/GmOvrlStMgrPer1/ApaIntv/Timer for ApaIntv/If Action Subsystem ==
  Action Port : ActionPort  ActionType=then
  Constant : Constant  Value=0  OutDataTypeStr=single
  CopyRight2 : Subsystem  Description=|  mask(Copyright Information){none=on}
      | Copyright info block.                                               
      |                                                                     
      | Place copyright information at the top of every subsystem in design.
      mask prompts: none "No parameters"
      mask help: Place copyright information at the top of every subsystem in design.
      mask Display:
      | NxtrConf = 'Nexteer Confidential';
      | 
      | sys = bdroot; %handle for the current model ("system")
      | first = get_param(sys,'Created');
      | first = first(end-3:end);  %year is last four digits
      | 
      | last = get_param(sys,'LastModifiedDate');
      | if isempty(last)
      |     last = datestr(now,'yyyy');
      | else
      |     last = last(end-3:end);
      | end
      | 
      | if strcmp(first,last)
      |     fprintf('%s -- Copyright %s Nexteer',NxtrConf,first)
      | else
      |     fprintf('%s -- %s%s- %s Nexteer',NxtrConf,char(169),first,last)
      | end
  Data Store Write : DataStoreWrite  DataStoreName=PrevApaIntvRefTi
  Data Type Conversion : DataTypeConversion  OutDataTypeStr=uint32
  GetRefTmr100MicroSec32bit : Subsystem
  Out : Outport
  wires:
  Constant/1 -> Data Type Conversion/1
  GetRefTmr100MicroSec32bit/1(RefTmr) -> Data Store Write/1
  Data Type Conversion/1 -> Out/1

== system CF009A_GmOvrlStMgr/GmOvrlStMgr/GmOvrlStMgrPer1/ApaIntv/Timer for ApaIntv/If Action Subsystem1 ==
  In1 : Inport
  Action Port : ActionPort  ActionType=else
  CopyRight2 : Subsystem  Description=|  mask(Copyright Information){none=on}
      | Copyright info block.                                               
      |                                                                     
      | Place copyright information at the top of every subsystem in design.
      mask prompts: none "No parameters"
      mask help: Place copyright information at the top of every subsystem in design.
      mask Display:
      | NxtrConf = 'Nexteer Confidential';
      | 
      | sys = bdroot; %handle for the current model ("system")
      | first = get_param(sys,'Created');
      | first = first(end-3:end);  %year is last four digits
      | 
      | last = get_param(sys,'LastModifiedDate');
      | if isempty(last)
      |     last = datestr(now,'yyyy');
      | else
      |     last = last(end-3:end);
      | end
      | 
      | if strcmp(first,last)
      |     fprintf('%s -- Copyright %s Nexteer',NxtrConf,first)
      | else
      |     fprintf('%s -- %s%s- %s Nexteer',NxtrConf,char(169),first,last)
      | end
  Out1 : Outport
  wires:
  In1/1 -> Out1/1
